simulink model "SingleTrack_RTW"  (Simulink 7.5)
settings: Solver=ode1  SolverMode=SingleTasking  StartTime=0.0  StopTime=inf  FixedStep=0.001  RelTol=1e-3
PreLoadFcn:
  | vehicle = 'Car'; if ~length(which('cmcmd')), cmenv; end
  | SingleTrack_RTW_bus;
  | SingleTrack_RTW_params;
InitFcn:
  | vehicle = 'Car'; if ~length(which('cmcmd')), cmenv; end
  | SingleTrack_RTW_bus;
  | SingleTrack_RTW_params;
values from neighbouring files (symbols this model uses):
  Car_Bdy1_mass = 650.0    (= 650)    [SingleTrack_RTW_params.m]    (also in UserVehicle_RTW_params.m)
  Car_Steering_i = 10.0    (= 10)    [SingleTrack_RTW_params.m]    (also in UserVehicle_RTW_params.m)
  Car_Whl_Radius = 0.31    [SingleTrack_RTW_params.m]    (also in UserVehicle_RTW_params.m)
  Car_WhlBaseF = 1.5    [SingleTrack_RTW_params.m]    (also in UserVehicle_RTW_params.m)
  Car_WhlBaseR = -1.5    [SingleTrack_RTW_params.m]    (also in UserVehicle_RTW_params.m)
  mEngineMax = 180    [SingleTrack_RTW_params.m]    (also in UserVehicle_RTW_params.m)
  PT_DL_iDiff = 4.1    [SingleTrack_RTW_params.m]    (also in UserVehicle_RTW_params.m)
  PT_GearBox_iForwardGears = [ 0 2.5 2.063 1.722 1.5 1.364 1.261]    [SingleTrack_RTW_params.m]    (also in UserVehicle_RTW_params.m)
libraries: CarMaker4SL x7
(part 3 of 3)

== system SingleTrack_RTW/SingleTrack/CreateBus Vhcl.Fr1/BdyFrame2Vhcl.Fr1A ==
  note: Translate pseudo BdyFrame interface to Vhcl.Fr1
  t_0 : Inport  OutDataType=sfix(16)  OutScaling=2^0
  v_0 : Inport  Port=2  OutDataType=sfix(16)  OutScaling=2^0
  a_0 : Inport  Port=3  OutDataType=sfix(16)  OutScaling=2^0
  omega_0 : Inport  Port=4  OutDataType=sfix(16)  OutScaling=2^0
  alpha_0 : Inport  Port=5  OutDataType=sfix(16)  OutScaling=2^0
  Tr2Fr0 : Inport  Port=6  OutDataType=sfix(16)  OutScaling=2^0
  Bus Creator : BusCreator  Inputs=24
  Demux{,1..3,5} (5 alike) : Demux  Outputs=3
  Demux4 : Demux  Outputs=9
  Vhcl.Fr1 : Outport  OutDataType=sfix(16)  OutScaling=2^0
  wires:
  Bus Creator/1 -> Vhcl.Fr1/1
  Demux/1 -> Bus Creator/1  "Vhcl Fr1 A_t_0 x"
  Demux/2 -> Bus Creator/2  "Vhcl Fr1A_t_0 y"
  Demux/3 -> Bus Creator/3  "Vhcl Fr1A_t_0 z"
  Demux1/1 -> Bus Creator/4  "Vhcl Fr1A_v_0 x"
  Demux1/2 -> Bus Creator/5  "Vhcl Fr1A_v_0 y"
  Demux1/3 -> Bus Creator/6  "Vhcl Fr1A_v_0 z"
  Demux2/1 -> Bus Creator/7  "Vhcl Fr1A_a_0 x"
  Demux2/2 -> Bus Creator/8  "Vhcl Fr1A_a_0 y"
  Demux2/3 -> Bus Creator/9  "Vhcl Fr1A_a_0 z"
  Demux3/1 -> Bus Creator/10  "Vhcl Fr1A_omega_0 x"
  Demux3/2 -> Bus Creator/11  "Vhcl Fr1A_omega_0 y"
  Demux3/3 -> Bus Creator/12  "Vhcl Fr1A_omega_0 z"
  Demux5/1 -> Bus Creator/13  "Vhcl Fr1A_alpha_0 x"
  Demux5/2 -> Bus Creator/14  "Vhcl Fr1A_alpha_0 y"
  Demux5/3 -> Bus Creator/15  "Vhcl Fr1A_alpha_0 z"
  Demux4/1 -> Bus Creator/16  "Vhcl Fr1A_Tr2Fr0 00"
  Demux4/2 -> Bus Creator/17  "Vhcl Fr1A_Tr2Fr0 01"
  Demux4/3 -> Bus Creator/18  "Vhcl Fr1A_Tr2Fr0 02"
  Demux4/4 -> Bus Creator/19  "Vhcl Fr1A_Tr2Fr0 10"
  Demux4/5 -> Bus Creator/20  "Vhcl Fr1A_Tr2Fr0 11"
  Demux4/6 -> Bus Creator/21  "Vhcl Fr1A_Tr2Fr0 12"
  Demux4/7 -> Bus Creator/22  "Vhcl Fr1A_Tr2Fr0 20"
  Demux4/8 -> Bus Creator/23  "Vhcl Fr1A_Tr2Fr0 21"
  Demux4/9 -> Bus Creator/24  "Vhcl Fr1A_Tr2Fr0 22"
  Tr2Fr0/1 -> Demux4/1
  alpha_0/1 -> Demux5/1
  omega_0/1 -> Demux3/1
  a_0/1 -> Demux2/1
  v_0/1 -> Demux1/1
  t_0/1 -> Demux/1

== system SingleTrack_RTW/SingleTrack/CreateBus Vhcl.Fr1/Tr2Fr0 ==
  Car : Inport  OutDataType=sfix(16)  OutScaling=2^0
  Bus Creator : BusCreator  Inputs=9
  Subsystem_00 : Subsystem
  Subsystem_01 : Subsystem
  Subsystem_02 : Subsystem
  Subsystem_10 : Subsystem
  Subsystem_11 : Subsystem
  Subsystem_12 : Subsystem
  Subsystem_20 : Subsystem
  Subsystem_21 : Subsystem
  Subsystem_22 : Subsystem
  sincos : Subsystem
  Tr2Fr0 : Outport  OutDataType=sfix(16)  OutScaling=2^0
  wires:
  Subsystem_12/1(Tr2Fr1_12) -> Bus Creator/6  "Tr2Fr1_12"
  Subsystem_11/1(Tr2Fr1_11) -> Bus Creator/5  "Tr2Fr1_11"
  Subsystem_02/1(Tr2Fr1_02) -> Bus Creator/3  "Tr2Fr0_02"
  Subsystem_01/1(Tr2Fr1_01) -> Bus Creator/2  "Tr2Fr0_01"
  Subsystem_22/1(Tr2Fr1_22) -> Bus Creator/9  "Tr2Fr0_22"
  Subsystem_21/1(Tr2Fr1_21) -> Bus Creator/8  "Tr2Fr0_21"
  Subsystem_20/1(Tr2Fr1_20) -> Bus Creator/7  "Tr2Fr0_20"
  Subsystem_10/1(Tr2Fr1_10) -> Bus Creator/4  "Tr2Fr0_10"
  Subsystem_00/1(Tr2Fr1_00) -> Bus Creator/1  "Tr2Fr0_00"
  Bus Creator/1 -> Tr2Fr0/1
  sincos/1(sincos) -> Subsystem_02/1(sincos), Subsystem_01/1(sincos), Subsystem_00/1(sincos), Subsystem_12/1(sincos), Subsystem_22/1(sincos), Subsystem_21/1(sincos), Subsystem_20/1(sincos), Subsystem_11/1(sincos), Subsystem_10/1(sincos)
  Car/1 -> sincos/1(Car)

== system SingleTrack_RTW/SingleTrack/CreateBus Vhcl.Fr1/a_0 ==
  Car : Inport  OutDataType=sfix(16)  OutScaling=2^0
  Tr2Fr0 : Inport  Port=2  OutDataType=sfix(16)  OutScaling=2^0
  Add : Sum  OutDataType=sfix(16)  OutScaling=2^-10
  Add1 : Sum  OutDataType=sfix(16)  OutScaling=2^-10
  Add2 : Sum  OutDataType=sfix(16)  OutScaling=2^-10
  Bus Selector1 : BusSelector  OutputSignals=Car_ax_1,Car_ay_1
  Bus Selector2 : BusSelector  OutputSignals=Tr2Fr0_00,Tr2Fr0_01,Tr2Fr0_10,Tr2Fr1_11,Tr2Fr0_20,Tr2Fr0_21
  Mux1 : Mux  Inputs=3
  Product{,1..5} (6 alike) : Product  OutDataType=sfix(16)  OutScaling=2^0  RndMeth=Zero
  a_0 : Outport  OutDataType=sfix(16)  OutScaling=2^0
  wires:
  Bus Selector2/5 -> Product5/2  "<Tr2Fr0_20>"
  Bus Selector2/6 -> Product4/2  "<Tr2Fr0_21>"
  Add2/1 -> Mux1/3
  Product4/1 -> Add2/2
  Product5/1 -> Add2/1
  Bus Selector2/4 -> Product2/2  "<Tr2Fr1_11>"
  Bus Selector2/3 -> Product3/2  "<Tr2Fr0_10>"
  Add1/1 -> Mux1/2
  Bus Selector2/2 -> Product/2  "<Tr2Fr0_01>"
  Bus Selector2/1 -> Product1/2  "<Tr2Fr0_00>"
  Product2/1 -> Add1/2
  Product3/1 -> Add1/1
  Add/1 -> Mux1/1
  Product/1 -> Add/2
  Product1/1 -> Add/1
  Bus Selector1/1 -> Product5/1, Product3/1, Product1/1  "<Car_ax_1>"
  Bus Selector1/2 -> Product4/1, Product2/1, Product/1  "<Car_ay_1>"
  Tr2Fr0/1 -> Bus Selector2/1
  Car/1 -> Bus Selector1/1
  Mux1/1 -> a_0/1

== system SingleTrack_RTW/SingleTrack/CreateBus Vhcl.Fr1/t_0 ==
  Car : Inport  OutDataType=sfix(16)  OutScaling=2^0
  Bus Selector : BusSelector  OutputSignals=Car_x,Car_y,Road_Fr1_z
  Mux : Mux  Inputs=3
  t_0 : Outport  OutDataType=sfix(16)  OutScaling=2^0
  wires:
  Mux/1 -> t_0/1
  Car/1 -> Bus Selector/1
  Bus Selector/3 -> Mux/3  "<Road_Fr1_z>"
  Bus Selector/2 -> Mux/2  "<Car_y>"
  Bus Selector/1 -> Mux/1  "<Car_x>"

== system SingleTrack_RTW/SingleTrack/CreateBus Vhcl.Fr1/v_0 ==
  Car : Inport  OutDataType=sfix(16)  OutScaling=2^0
  Tr2Fr0 : Inport  Port=2  OutDataType=sfix(16)  OutScaling=2^0
  Bus Selector1 : BusSelector  OutputSignals=Car_vx_1
  Bus Selector2 : BusSelector  OutputSignals=Tr2Fr0_00,Tr2Fr0_10,Tr2Fr0_20
  Mux1 : Mux  Inputs=3
  Product : Product  OutDataType=sfix(16)  OutScaling=2^0  RndMeth=Zero
  Product1 : Product  OutDataType=sfix(16)  OutScaling=2^0  RndMeth=Zero
  Product2 : Product  OutDataType=sfix(16)  OutScaling=2^0  RndMeth=Zero
  v_0 : Outport  OutDataType=sfix(16)  OutScaling=2^0
  wires:
  Product2/1 -> Mux1/3
  Product1/1 -> Mux1/2
  Product/1 -> Mux1/1
  Bus Selector1/1 -> Product2/1, Product1/1, Product/1  "<Car_vx_1>"
  Bus Selector2/3 -> Product2/2  "<Tr2Fr0_20>"
  Bus Selector2/2 -> Product1/2  "<Tr2Fr0_10>"
  Bus Selector2/1 -> Product/2  "<Tr2Fr0_00>"
  Tr2Fr0/1 -> Bus Selector2/1
  Mux1/1 -> v_0/1
  Car/1 -> Bus Selector1/1

== system SingleTrack_RTW/SingleTrack/single-track mass point model/Car.v_1 ==
  ax : Inport
  Constant1 : Constant  Value=0.1  OutDataType=sfix(16)  OutScaling=2^0
  PassIfSim : Subsystem
  Read CM Parameter : CarMaker4SL/Read CM Parameter  xfile=Testrun  xkey=DrivMan.Init.Velocity  xnout=1  xdefaults=0  xmuxed=on
  kmh2ms : Gain  Gain=1000/3600  ParameterDataType=sfix(16)  ParameterScaling=2^0  OutDataType=sfix(16)  OutScaling=2^0  OutDataTypeStr=Inherit: Inherit via back propagation  SaturateOnIntegerOverflow=on  ParamDataTypeStr=Inherit: Same as input
  vMin : MinMax  Function=max  Inputs=2  OutDataType=sfix(16)  OutScaling=2^0  SaturateOnIntegerOverflow=on  InputSameDT=on
  v_dot * dt : Integrator  ExternalReset=level  InitialConditionSource=external  InitialCondition=22.222
  v_1 : Outport  PortDimensions=1
  wires:
  PassIfSim/1(Out1) -> v_dot * dt/1
  ax/1 -> PassIfSim/1(In1)
  v_dot * dt/1 -> v_1/1
  vMin/1 -> v_dot * dt/3
  [TRStart] -> v_dot * dt/2
  Constant1/1 -> vMin/1
  kmh2ms/1 -> vMin/2
  Read CM Parameter/1 -> kmh2ms/1

== system SingleTrack_RTW/SingleTrack/single-track mass point model/PassIfSim ==
  note: Output original value only when simulating,
      | and zero during pre- or postprocessing.
  In1 : Inport  OutDataType=sfix(16)  OutScaling=2^0
  "   " : Product  OutDataType=sfix(16)  OutScaling=2^0  SaturateOnIntegerOverflow=on  InputSameDT=on  OutDataTypeStr=Inherit: Same as first input
  Data Type Conversion : DataTypeConversion  OutDataType=sfix(16)  OutScaling=2^0
  Out1 : Outport  OutDataType=sfix(16)  OutScaling=2^0
  wires:
  In1/1 -> "   "/1
  Data Type Conversion/1 -> "   "/2
  "   "/1 -> Out1/1
  [TRSim] -> Data Type Conversion/1

== system SingleTrack_RTW/SingleTrack/single-track mass point model/PassIfSim1 ==
  note: Output original value only when simulating,
      | and zero during pre- or postprocessing.
  In1 : Inport  OutDataType=sfix(16)  OutScaling=2^0
  "   " : Product  OutDataType=sfix(16)  OutScaling=2^0  SaturateOnIntegerOverflow=on  InputSameDT=on  OutDataTypeStr=Inherit: Same as first input
  Data Type Conversion : DataTypeConversion  OutDataType=sfix(16)  OutScaling=2^0
  Out1 : Outport  OutDataType=sfix(16)  OutScaling=2^0
  wires:
  In1/1 -> "   "/1
  Data Type Conversion/1 -> "   "/2
  "   "/1 -> Out1/1
  [TRSim] -> Data Type Conversion/1

== system SingleTrack_RTW/SingleTrack/single-track mass point model/PassIfSim2 ==
  note: Output original value only when simulating,
      | and zero during pre- or postprocessing.
  In1 : Inport  OutDataType=sfix(16)  OutScaling=2^0
  "   " : Product  OutDataType=sfix(16)  OutScaling=2^0  SaturateOnIntegerOverflow=on  InputSameDT=on  OutDataTypeStr=Inherit: Same as first input
  Data Type Conversion : DataTypeConversion  OutDataType=sfix(16)  OutScaling=2^0
  Out1 : Outport  OutDataType=sfix(16)  OutScaling=2^0
  wires:
  In1/1 -> "   "/1
  Data Type Conversion/1 -> "   "/2
  "   "/1 -> Out1/1
  [TRSim] -> Data Type Conversion/1

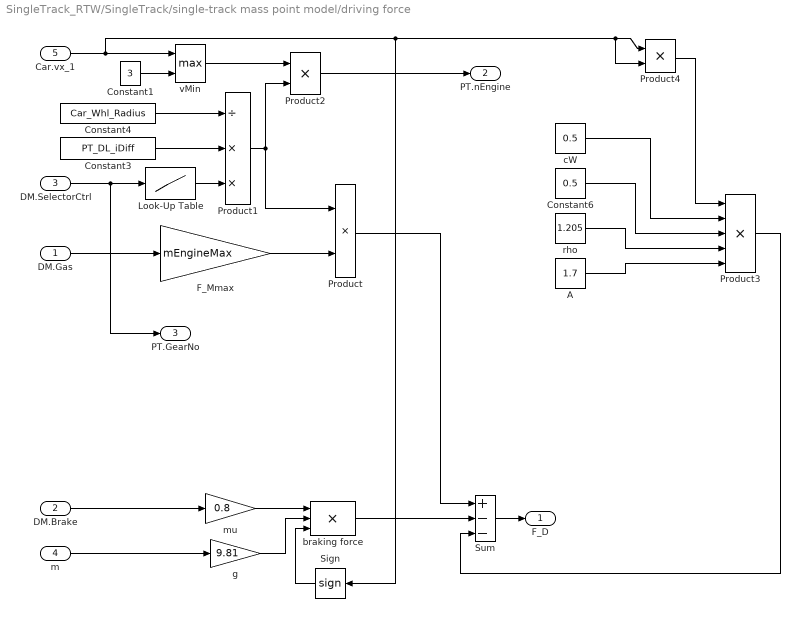
== system SingleTrack_RTW/SingleTrack/single-track mass point model/driving force ==
  DM.Gas : Inport  OutDataType=sfix(16)  OutScaling=2^0
  DM.Brake : Inport  Port=2  OutDataType=sfix(16)  OutScaling=2^0
  DM.SelectorCtrl : Inport  Port=3  OutDataType=sfix(16)  OutScaling=2^0
  m : Inport  Port=4  OutDataType=sfix(16)  OutScaling=2^0
  Car.vx_1 : Inport  Port=5  OutDataType=sfix(16)  OutScaling=2^0
  A : Constant  Value=1.7  OutDataType=sfix(16)  OutScaling=2^0
  Constant1 : Constant  Value=3  OutDataType=sfix(16)  OutScaling=2^0
  Constant3 : Constant  Value=PT_DL_iDiff  OutDataType=sfix(16)  OutScaling=2^0
  Constant4 : Constant  Value=Car_Whl_Radius  OutDataType=sfix(16)  OutScaling=2^0
  Constant6 : Constant  Value=0.5  OutDataType=sfix(16)  OutScaling=2^0
  "F_Mmax " : Gain  Gain=mEngineMax  ParameterDataType=sfix(16)  ParameterScaling=2^0  OutDataType=sfix(16)  OutScaling=2^0  SaturateOnIntegerOverflow=on  OutDataTypeStr=Inherit: Same as input  ParamDataTypeStr=Inherit: Same as input
  Look-Up Table : Lookup  InputValues=[0 1 2 3 4 5 6]  Table=PT_GearBox_iForwardGears  LookUpMeth=Interpolation-Use End Values  OutDataType=sfix(16)  OutScaling=2^0  SaturateOnIntegerOverflow=on
  Product : Product  Inputs=**  OutDataType=sfix(16)  OutScaling=2^0  SaturateOnIntegerOverflow=on  InputSameDT=on  OutDataTypeStr=Inherit: Same as first input
  Product1 : Product  Inputs=/**  OutDataType=sfix(16)  OutScaling=2^0  SaturateOnIntegerOverflow=on  InputSameDT=on  OutDataTypeStr=Inherit: Same as first input
  Product2 : Product  OutDataType=sfix(16)  OutScaling=2^0  SaturateOnIntegerOverflow=on  InputSameDT=on  OutDataTypeStr=Inherit: Same as first input
  Product3 : Product  Inputs=5  OutDataType=sfix(16)  OutScaling=2^0  SaturateOnIntegerOverflow=on  InputSameDT=on  OutDataTypeStr=Inherit: Same as first input
  Product4 : Product  OutDataType=sfix(16)  OutScaling=2^0  SaturateOnIntegerOverflow=on  InputSameDT=on  OutDataTypeStr=Inherit: Same as first input
  Sign : Signum
  Sum : Sum  Inputs=+--  OutDataType=sfix(16)  OutScaling=2^0  SaturateOnIntegerOverflow=on  InputSameDT=on  OutDataTypeStr=Inherit: Same as first input
  braking force : Product  Inputs=3  OutDataType=sfix(16)  OutScaling=2^0  SaturateOnIntegerOverflow=on  InputSameDT=on  OutDataTypeStr=Inherit: Same as first input
  cW : Constant  Value=0.5  OutDataType=sfix(16)  OutScaling=2^0
  g : Gain  Gain=9.81  ParameterDataType=sfix(16)  ParameterScaling=2^0  OutDataType=sfix(16)  OutScaling=2^0  SaturateOnIntegerOverflow=on  OutDataTypeStr=Inherit: Same as input  ParamDataTypeStr=Inherit: Same as input
  mu : Gain  Gain=0.8  ParameterDataType=sfix(16)  ParameterScaling=2^0  OutDataType=sfix(16)  OutScaling=2^0  SaturateOnIntegerOverflow=on  OutDataTypeStr=Inherit: Same as input  ParamDataTypeStr=Inherit: Same as input
  rho : Constant  Value=1.205  OutDataType=sfix(16)  OutScaling=2^0
  vMin : MinMax  Function=max  Inputs=2  OutDataType=sfix(16)  OutScaling=2^0  SaturateOnIntegerOverflow=on  InputSameDT=on
  F_D : Outport  OutDataType=sfix(16)  OutScaling=2^0
  PT.nEngine : Outport  Port=2  OutDataType=sfix(16)  OutScaling=2^0
  PT.GearNo : Outport  Port=3  OutDataType=sfix(16)  OutScaling=2^0
  wires:
  vMin/1 -> Product2/1
  Car.vx_1/1 -> vMin/1, Product4/1, Product4/2, Sign/1
  Constant1/1 -> vMin/2
  DM.Brake/1 -> mu/1
  "F_Mmax "/1 -> Product/2
  Product2/1 -> PT.nEngine/1
  Look-Up Table/1 -> Product1/3
  Product1/1 -> Product/1, Product2/2
  Constant4/1 -> Product1/1
  Constant3/1 -> Product1/2
  Product/1 -> Sum/1
  Sum/1 -> F_D/1
  braking force/1 -> Sum/2
  g/1 -> braking force/2
  m/1 -> g/1
  mu/1 -> braking force/1
  DM.Gas/1 -> "F_Mmax "/1
  A/1 -> Product3/5
  rho/1 -> Product3/4
  Constant6/1 -> Product3/3
  cW/1 -> Product3/2
  Product4/1 -> Product3/1
  Product3/1 -> Sum/3
  Sign/1 -> braking force/3
  DM.SelectorCtrl/1 -> Look-Up Table/1, PT.GearNo/1

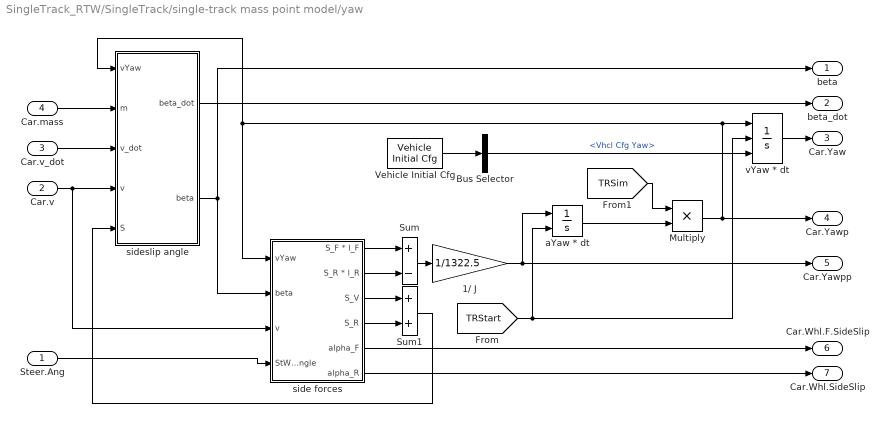
== system SingleTrack_RTW/SingleTrack/single-track mass point model/yaw ==
  Steer.Ang : Inport  OutDataType=sfix(16)  OutScaling=2^0
  Car.v : Inport  Port=2  OutDataType=sfix(16)  OutScaling=2^0
  Car.v_dot : Inport  Port=3  OutDataType=sfix(16)  OutScaling=2^0
  Car.mass : Inport  Port=4  OutDataType=sfix(16)  OutScaling=2^0
  1/ J : Gain  Gain=1/1322.5  ParameterDataType=sfix(16)  ParameterScaling=2^0  OutDataType=sfix(16)  OutScaling=2^0  SaturateOnIntegerOverflow=on  OutDataTypeStr=Inherit: Same as input  ParamDataTypeStr=Inherit: Same as input
  Bus Selector : BusSelector  OutputSignals=Vhcl Cfg Yaw
  Multiply : Product  Inputs=**  OutDataTypeMode=double  OutDataType=sfix(16)  OutScaling=2^-10  OutDataTypeStr=double
  Sum : Sum  Inputs=+-  OutDataType=sfix(16)  OutScaling=2^0  SaturateOnIntegerOverflow=on  InputSameDT=on  OutDataTypeStr=Inherit: Same as first input
  Sum1 : Sum  OutDataType=sfix(16)  OutScaling=2^0  SaturateOnIntegerOverflow=on  InputSameDT=on  OutDataTypeStr=Inherit: Same as first input
  Vehicle Initial Cfg : CarMaker4SL/Vehicle Initial Cfg  SystemSampleTime=-1
  aYaw * dt : Integrator  ExternalReset=level
  side forces : Subsystem
  sideslip angle : Subsystem
  vYaw * dt : Integrator  ExternalReset=level  InitialConditionSource=external
  beta : Outport  OutDataType=sfix(16)  OutScaling=2^0
  beta_dot : Outport  Port=2  OutDataType=sfix(16)  OutScaling=2^0
  Car.Yaw : Outport  Port=3  OutDataType=sfix(16)  OutScaling=2^0
  Car.Yawp : Outport  Port=4  OutDataType=sfix(16)  OutScaling=2^0
  Car.Yawpp : Outport  Port=5  OutDataType=sfix(16)  OutScaling=2^0
  Car.Whl.F.SideSlip : Outport  Port=6  OutDataType=sfix(16)  OutScaling=2^0
  Car.Whl.SideSlip : Outport  Port=7  OutDataType=sfix(16)  OutScaling=2^0
  wires:
  Bus Selector/1 -> vYaw * dt/3  "<Vhcl Cfg Yaw>"
  side forces/6(alpha_R) -> Car.Whl.SideSlip/1
  side forces/5(alpha_F) -> Car.Whl.F.SideSlip/1
  sideslip angle/1(beta_dot) -> beta_dot/1
  Steer.Ang/1 -> side forces/4(StWhlAngle)
  sideslip angle/2(beta) -> beta/1, side forces/2(beta)
  Car.mass/1 -> sideslip angle/2(m)
  Car.v_dot/1 -> sideslip angle/3(v_dot)
  Sum1/1 -> sideslip angle/5(S)
  Sum/1 -> 1/ J/1
  side forces/1(S_F * l_F) -> Sum/1
  side forces/2(S_R * l_R) -> Sum/2
  1/ J/1 -> Car.Yawpp/1, aYaw * dt/1
  side forces/3(S_V) -> Sum1/1
  side forces/4(S_R) -> Sum1/2
  Car.v/1 -> sideslip angle/4(v), side forces/3(v)
  vYaw * dt/1 -> Car.Yaw/1
  Multiply/1 -> side forces/1(vYaw), sideslip angle/1(vYaw), vYaw * dt/1, Car.Yawp/1
  [TRStart] -> vYaw * dt/2, aYaw * dt/2
  aYaw * dt/1 -> Multiply/2
  [TRSim] -> Multiply/1
  Vehicle Initial Cfg/1 -> Bus Selector/1

== system SingleTrack_RTW/SingleTrack/CreateBus Vhcl.Fr1/Tr2Fr0/Subsystem_00 ==
  sincos : Inport  OutDataType=sfix(16)  OutScaling=2^0
  Bus Selector : BusSelector  OutputSignals=cry,crz
  Product : Product  OutDataType=sfix(16)  OutScaling=2^0  RndMeth=Zero
  Tr2Fr1_00 : Outport  OutDataType=sfix(16)  OutScaling=2^0
  wires:
  Bus Selector/2 -> Product/2  "<crz>"
  Bus Selector/1 -> Product/1  "<cry>"
  Product/1 -> Tr2Fr1_00/1
  sincos/1 -> Bus Selector/1

== system SingleTrack_RTW/SingleTrack/CreateBus Vhcl.Fr1/Tr2Fr0/Subsystem_01 ==
  sincos : Inport  OutDataType=sfix(16)  OutScaling=2^0
  Add : Sum  Inputs=+-  OutDataType=sfix(16)  OutScaling=2^-10
  Bus Selector : BusSelector  OutputSignals=srx,sry,crz,crx,srz
  Product : Product  Inputs=3  OutDataType=sfix(16)  OutScaling=2^0  RndMeth=Zero
  Product1 : Product  OutDataType=sfix(16)  OutScaling=2^0  RndMeth=Zero
  Tr2Fr1_01 : Outport  OutDataType=sfix(16)  OutScaling=2^0
  wires:
  Bus Selector/5 -> Product1/2  "<srz>"
  Bus Selector/4 -> Product1/1  "<crx>"
  Bus Selector/3 -> Product/3  "<crz>"
  Bus Selector/2 -> Product/2  "<sry>"
  Bus Selector/1 -> Product/1  "<srx>"
  Add/1 -> Tr2Fr1_01/1
  Product1/1 -> Add/2
  Product/1 -> Add/1
  sincos/1 -> Bus Selector/1

== system SingleTrack_RTW/SingleTrack/CreateBus Vhcl.Fr1/Tr2Fr0/Subsystem_02 ==
  sincos : Inport  OutDataType=sfix(16)  OutScaling=2^0
  Add : Sum  OutDataType=sfix(16)  OutScaling=2^-10
  Bus Selector : BusSelector  OutputSignals=crx,sry,crz,srx,srz
  Product : Product  Inputs=3  OutDataType=sfix(16)  OutScaling=2^0  RndMeth=Zero
  Product1 : Product  OutDataType=sfix(16)  OutScaling=2^0  RndMeth=Zero
  Tr2Fr1_02 : Outport  OutDataType=sfix(16)  OutScaling=2^0
  wires:
  Bus Selector/4 -> Product1/1  "<srx>"
  Bus Selector/5 -> Product1/2  "<srz>"
  Bus Selector/3 -> Product/3  "<crz>"
  Bus Selector/2 -> Product/2  "<sry>"
  Bus Selector/1 -> Product/1  "<crx>"
  sincos/1 -> Bus Selector/1
  Product/1 -> Add/1
  Product1/1 -> Add/2
  Add/1 -> Tr2Fr1_02/1

== system SingleTrack_RTW/SingleTrack/CreateBus Vhcl.Fr1/Tr2Fr0/Subsystem_10 ==
  sincos : Inport  OutDataType=sfix(16)  OutScaling=2^0
  Bus Selector : BusSelector  OutputSignals=cry,srz
  Product : Product  OutDataType=sfix(16)  OutScaling=2^0  RndMeth=Zero
  Tr2Fr1_10 : Outport  OutDataType=sfix(16)  OutScaling=2^0
  wires:
  sincos/1 -> Bus Selector/1
  Product/1 -> Tr2Fr1_10/1
  Bus Selector/1 -> Product/1  "<cry>"
  Bus Selector/2 -> Product/2  "<srz>"

== system SingleTrack_RTW/SingleTrack/CreateBus Vhcl.Fr1/Tr2Fr0/Subsystem_11 ==
  sincos : Inport  OutDataType=sfix(16)  OutScaling=2^0
  Add : Sum  OutDataType=sfix(16)  OutScaling=2^-10
  Bus Selector : BusSelector  OutputSignals=srx,sry,srz,crx,crz
  Product : Product  Inputs=3  OutDataType=sfix(16)  OutScaling=2^0  RndMeth=Zero
  Product1 : Product  OutDataType=sfix(16)  OutScaling=2^0  RndMeth=Zero
  Tr2Fr1_11 : Outport  OutDataType=sfix(16)  OutScaling=2^0
  wires:
  Bus Selector/4 -> Product1/1  "<crx>"
  Bus Selector/5 -> Product1/2  "<crz>"
  Bus Selector/3 -> Product/3  "<srz>"
  Bus Selector/2 -> Product/2  "<sry>"
  Bus Selector/1 -> Product/1  "<srx>"
  Add/1 -> Tr2Fr1_11/1
  Product1/1 -> Add/2
  Product/1 -> Add/1
  sincos/1 -> Bus Selector/1

== system SingleTrack_RTW/SingleTrack/CreateBus Vhcl.Fr1/Tr2Fr0/Subsystem_12 ==
  sincos : Inport  OutDataType=sfix(16)  OutScaling=2^0
  Add : Sum  Inputs=+-  OutDataType=sfix(16)  OutScaling=2^-10
  Bus Selector : BusSelector  OutputSignals=crx,sry,srz,srx,crz
  Product : Product  Inputs=3  OutDataType=sfix(16)  OutScaling=2^0  RndMeth=Zero
  Product1 : Product  OutDataType=sfix(16)  OutScaling=2^0  RndMeth=Zero
  Tr2Fr1_12 : Outport  OutDataType=sfix(16)  OutScaling=2^0
  wires:
  Bus Selector/4 -> Product1/1  "<srx>"
  Bus Selector/5 -> Product1/2  "<crz>"
  Bus Selector/3 -> Product/3  "<srz>"
  Bus Selector/2 -> Product/2  "<sry>"
  Bus Selector/1 -> Product/1  "<crx>"
  sincos/1 -> Bus Selector/1
  Product/1 -> Add/1
  Product1/1 -> Add/2
  Add/1 -> Tr2Fr1_12/1

== system SingleTrack_RTW/SingleTrack/CreateBus Vhcl.Fr1/Tr2Fr0/Subsystem_20 ==
  sincos : Inport  OutDataType=sfix(16)  OutScaling=2^0
  Bus Selector : BusSelector  OutputSignals=sry
  Gain : Gain  Gain=-1  ParameterDataType=sfix(16)  ParameterScaling=2^0  OutDataType=sfix(16)  OutScaling=2^0
  Tr2Fr1_20 : Outport  OutDataType=sfix(16)  OutScaling=2^0
  wires:
  Bus Selector/1 -> Gain/1  "<sry>"
  Gain/1 -> Tr2Fr1_20/1
  sincos/1 -> Bus Selector/1

== system SingleTrack_RTW/SingleTrack/CreateBus Vhcl.Fr1/Tr2Fr0/Subsystem_21 ==
  sincos : Inport  OutDataType=sfix(16)  OutScaling=2^0
  Bus Selector : BusSelector  OutputSignals=srx,cry
  Product : Product  OutDataType=sfix(16)  OutScaling=2^0  RndMeth=Zero
  Tr2Fr1_21 : Outport  OutDataType=sfix(16)  OutScaling=2^0
  wires:
  Bus Selector/2 -> Product/2  "<cry>"
  Bus Selector/1 -> Product/1  "<srx>"
  Product/1 -> Tr2Fr1_21/1
  sincos/1 -> Bus Selector/1

== system SingleTrack_RTW/SingleTrack/CreateBus Vhcl.Fr1/Tr2Fr0/Subsystem_22 ==
  sincos : Inport  OutDataType=sfix(16)  OutScaling=2^0
  Bus Selector : BusSelector  OutputSignals=crx,cry
  Product : Product  OutDataType=sfix(16)  OutScaling=2^0  RndMeth=Zero
  Tr2Fr1_22 : Outport  OutDataType=sfix(16)  OutScaling=2^0
  wires:
  Bus Selector/2 -> Product/2  "<cry>"
  Bus Selector/1 -> Product/1  "<crx>"
  sincos/1 -> Bus Selector/1
  Product/1 -> Tr2Fr1_22/1

== system SingleTrack_RTW/SingleTrack/CreateBus Vhcl.Fr1/Tr2Fr0/sincos ==
  Car : Inport  OutDataType=sfix(16)  OutScaling=2^0
  Bus Creator : BusCreator  Inputs=6
  Bus Selector : BusSelector  OutputSignals=Road_Fr1_rx,Road_Fr1_ry,Car_Yaw
  Trigonometric Function : Trigonometry
  Trigonometric Function1 : Trigonometry  Operator=cos
  Trigonometric Function2 : Trigonometry
  Trigonometric Function3 : Trigonometry
  Trigonometric Function4 : Trigonometry  Operator=cos
  Trigonometric Function5 : Trigonometry  Operator=cos
  sincos : Outport  OutDataType=sfix(16)  OutScaling=2^0
  wires:
  Bus Creator/1 -> sincos/1
  Trigonometric Function/1 -> Bus Creator/1  "srx"
  Trigonometric Function3/1 -> Bus Creator/2  "sry"
  Trigonometric Function2/1 -> Bus Creator/3  "srz"
  Trigonometric Function1/1 -> Bus Creator/4  "crx"
  Trigonometric Function4/1 -> Bus Creator/5  "cry"
  Trigonometric Function5/1 -> Bus Creator/6  "crz"
  Car/1 -> Bus Selector/1
  Bus Selector/3 -> Trigonometric Function5/1, Trigonometric Function2/1  "<Car_Yaw>"
  Bus Selector/2 -> Trigonometric Function4/1, Trigonometric Function3/1  "<Road_Fr1_ry>"
  Bus Selector/1 -> Trigonometric Function1/1, Trigonometric Function/1  "<Road_Fr1_rx>"

== system SingleTrack_RTW/SingleTrack/single-track mass point model/Car.v_1/PassIfSim ==
  note: Output original value only when simulating,
      | and zero during pre- or postprocessing.
  In1 : Inport  OutDataType=sfix(16)  OutScaling=2^0
  "   " : Product  OutDataType=sfix(16)  OutScaling=2^0  SaturateOnIntegerOverflow=on  InputSameDT=on  OutDataTypeStr=Inherit: Same as first input
  Data Type Conversion : DataTypeConversion  OutDataType=sfix(16)  OutScaling=2^0
  Out1 : Outport  OutDataType=sfix(16)  OutScaling=2^0
  wires:
  In1/1 -> "   "/1
  Data Type Conversion/1 -> "   "/2
  "   "/1 -> Out1/1
  [TRSim] -> Data Type Conversion/1

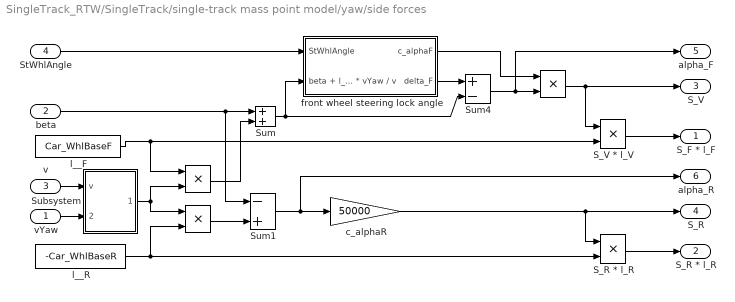
== system SingleTrack_RTW/SingleTrack/single-track mass point model/yaw/side forces ==
  vYaw : Inport  OutDataType=sfix(16)  OutScaling=2^0
  beta : Inport  Port=2  OutDataType=sfix(16)  OutScaling=2^0
  v : Inport  Port=3  OutDataType=sfix(16)  OutScaling=2^0
  StWhlAngle : Inport  Port=4  OutDataType=sfix(16)  OutScaling=2^0
  " " : Product  OutDataType=sfix(16)  OutScaling=2^0  SaturateOnIntegerOverflow=on  InputSameDT=on  OutDataTypeStr=Inherit: Same as first input
  "  " : Product  OutDataType=sfix(16)  OutScaling=2^0  SaturateOnIntegerOverflow=on  InputSameDT=on  OutDataTypeStr=Inherit: Same as first input
  "            " : Product  OutDataType=sfix(16)  OutScaling=2^0  SaturateOnIntegerOverflow=on  InputSameDT=on  OutDataTypeStr=Inherit: Same as first input
  "S_R * l_R " : Product  OutDataType=sfix(16)  OutScaling=2^0  SaturateOnIntegerOverflow=on  InputSameDT=on  OutDataTypeStr=Inherit: Same as first input
  "S_V * l_V " : Product  OutDataType=sfix(16)  OutScaling=2^0  SaturateOnIntegerOverflow=on  InputSameDT=on  OutDataTypeStr=Inherit: Same as first input
  Subsystem : Subsystem
  Sum : Sum  OutDataType=sfix(16)  OutScaling=2^0  SaturateOnIntegerOverflow=on  InputSameDT=on  OutDataTypeStr=Inherit: Same as first input
  Sum1 : Sum  Inputs=-+  OutDataType=sfix(16)  OutScaling=2^0  SaturateOnIntegerOverflow=on  InputSameDT=on  OutDataTypeStr=Inherit: Same as first input
  Sum4 : Sum  Inputs=+-  OutDataType=sfix(16)  OutScaling=2^0  SaturateOnIntegerOverflow=on  InputSameDT=on  OutDataTypeStr=Inherit: Same as first input
  c_alphaR : Gain  Gain=50000  ParameterDataType=sfix(16)  ParameterScaling=2^0  OutDataType=sfix(16)  OutScaling=2^0  SaturateOnIntegerOverflow=on  OutDataTypeStr=Inherit: Same as input  ParamDataTypeStr=Inherit: Same as input
  front wheel steering lock angle : Subsystem
  l__F : Constant  Value=Car_WhlBaseF  OutDataType=sfix(16)  OutScaling=2^0
  l__R : Constant  Value=-Car_WhlBaseR  OutDataType=sfix(16)  OutScaling=2^0
  S_F * l_F : Outport  OutDataType=sfix(16)  OutScaling=2^0
  S_R * l_R : Outport  Port=2  OutDataType=sfix(16)  OutScaling=2^0
  S_V : Outport  Port=3  OutDataType=sfix(16)  OutScaling=2^0
  S_R : Outport  Port=4  OutDataType=sfix(16)  OutScaling=2^0
  alpha_F : Outport  Port=5  OutDataType=sfix(16)  OutScaling=2^0
  alpha_R : Outport  Port=6  OutDataType=sfix(16)  OutScaling=2^0
  wires:
  front wheel steering lock angle/1(c_alphaF) -> "            "/1
  StWhlAngle/1 -> front wheel steering lock angle/1(StWhlAngle)
  "S_R * l_R "/1 -> S_R * l_R/1
  Sum4/1 -> alpha_F/1, "            "/2
  front wheel steering lock angle/2(delta_F) -> Sum4/1
  Sum/1 -> front wheel steering lock angle/2(beta + l_F * vYaw / v), Sum4/2
  v/1 -> Subsystem/1(v)
  vYaw/1 -> Subsystem/2(vYaw)
  "S_V * l_V "/1 -> S_F * l_F/1
  "            "/1 -> S_V/1, "S_V * l_V "/1
  c_alphaR/1 -> S_R/1, "S_R * l_R "/1
  Sum1/1 -> alpha_R/1, c_alphaR/1
  "  "/1 -> Sum/2
  " "/1 -> Sum1/2
  l__R/1 -> "S_R * l_R "/2, " "/2
  Subsystem/1(vYaw/v) -> "  "/2, " "/1
  l__F/1 -> "S_V * l_V "/2, "  "/1
  beta/1 -> Sum/1, Sum1/1

== system SingleTrack_RTW/SingleTrack/single-track mass point model/yaw/sideslip angle ==
  vYaw : Inport  OutDataType=sfix(16)  OutScaling=2^0
  m : Inport  Port=2  OutDataType=sfix(16)  OutScaling=2^0
  v_dot : Inport  Port=3  OutDataType=sfix(16)  OutScaling=2^0
  v : Inport  Port=4  OutDataType=sfix(16)  OutScaling=2^0
  S : Inport  Port=5  OutDataType=sfix(16)  OutScaling=2^0
  " " : Product  Inputs=*/  OutDataType=sfix(16)  OutScaling=2^0  SaturateOnIntegerOverflow=on  InputSameDT=on  OutDataTypeStr=Inherit: Same as first input
  "  " : Product  OutDataType=sfix(16)  OutScaling=2^0  SaturateOnIntegerOverflow=on  InputSameDT=on  OutDataTypeStr=Inherit: Same as first input
  Subsystem : Subsystem
  Sum2 : Sum  Inputs=+-  OutDataType=sfix(16)  OutScaling=2^0  SaturateOnIntegerOverflow=on  InputSameDT=on  OutDataTypeStr=Inherit: Same as first input
  beta_dot * dt : Integrator  ExternalReset=level
  beta_dot : Outport  OutDataType=sfix(16)  OutScaling=2^0
  beta : Outport  Port=2  OutDataType=sfix(16)  OutScaling=2^0
  wires:
  v/1 -> Subsystem/2(v)
  Subsystem/1(Out1) -> beta_dot/1, beta_dot * dt/1
  vYaw/1 -> Subsystem/1(vYaw)
  Sum2/1 -> Subsystem/3(In3)
  "  "/1 -> Sum2/2
  m/1 -> " "/2
  v_dot/1 -> "  "/1
  " "/1 -> Sum2/1
  S/1 -> " "/1
  beta_dot * dt/1 -> "  "/2, beta/1
  [TRStart] -> beta_dot * dt/2

== system SingleTrack_RTW/SingleTrack/single-track mass point model/yaw/side forces/Subsystem ==
  v : Inport
  vYaw : Inport  Port=2
  If : If  IfExpression=u1 > 0.1 | u1 < -0.1
  If Action Subsystem : Subsystem  TreatAsAtomicUnit=on
  If Action Subsystem1 : Subsystem  TreatAsAtomicUnit=on
  Merge : Merge  InitialOutput=0
  vYaw/v : Outport
  wires:
  v/1 -> If Action Subsystem/1(v), If/1
  vYaw/1 -> If Action Subsystem/2(vYaw)
  If/1 -> If Action Subsystem/Action
  If/2 -> If Action Subsystem1/Action
  Merge/1 -> vYaw/v/1
  If Action Subsystem/1(Out1) -> Merge/1
  If Action Subsystem1/1(Out1) -> Merge/2

== system SingleTrack_RTW/SingleTrack/single-track mass point model/yaw/side forces/front wheel steering lock angle ==
  StWhlAngle : Inport  OutDataType=sfix(16)  OutScaling=2^0
  beta + l_F * vYaw / v : Inport  Port=2  OutDataType=sfix(16)  OutScaling=2^0
  "   " : Product  OutDataType=sfix(16)  OutScaling=2^0  SaturateOnIntegerOverflow=on  InputSameDT=on  OutDataTypeStr=Inherit: Same as first input
  "     " : Constant  OutDataType=sfix(16)  OutScaling=2^0
  "      " : Product  Inputs=*/  OutDataType=sfix(16)  OutScaling=2^0  SaturateOnIntegerOverflow=on  InputSameDT=on  OutDataTypeStr=Inherit: Same as first input
  "       " : Product  Inputs=*/*  OutDataType=sfix(16)  OutScaling=2^0  SaturateOnIntegerOverflow=on  InputSameDT=on  OutDataTypeStr=Inherit: Same as first input
  1/ i_S : Gain  Gain=1/Car_Steering_i  ParameterDataType=sfix(16)  ParameterScaling=2^0  OutDataType=sfix(16)  OutScaling=2^0  SaturateOnIntegerOverflow=on  OutDataTypeStr=Inherit: Same as input  ParamDataTypeStr=Inherit: Same as input
  C_S : Constant  Value=10000  OutDataType=sfix(16)  OutScaling=2^0
  Sum2 : Sum  OutDataType=sfix(16)  OutScaling=2^0  SaturateOnIntegerOverflow=on  InputSameDT=on  OutDataTypeStr=Inherit: Same as first input
  Sum3 : Sum  OutDataType=sfix(16)  OutScaling=2^0  SaturateOnIntegerOverflow=on  InputSameDT=on  OutDataTypeStr=Inherit: Same as first input
  "c_alphaF " : Constant  Value=50000  OutDataType=sfix(16)  OutScaling=2^0
  n_F : Constant  Value=0.06  OutDataType=sfix(16)  OutScaling=2^0
  c_alphaF : Outport  OutDataType=sfix(16)  OutScaling=2^0
  delta_F : Outport  Port=2  OutDataType=sfix(16)  OutScaling=2^0
  wires:
  "      "/1 -> delta_F/1
  "c_alphaF "/1 -> "       "/1, c_alphaF/1
  n_F/1 -> "       "/3
  C_S/1 -> "       "/2
  Sum2/1 -> "      "/1
  Sum3/1 -> "      "/2
  "     "/1 -> Sum3/1
  1/ i_S/1 -> Sum2/1
  "   "/1 -> Sum2/2
  StWhlAngle/1 -> 1/ i_S/1
  "       "/1 -> "   "/1, Sum3/2
  beta + l_F * vYaw / v/1 -> "   "/2

== system SingleTrack_RTW/SingleTrack/single-track mass point model/yaw/sideslip angle/Subsystem ==
  vYaw : Inport
  v : Inport  Port=2
  In3 : Inport  Port=3
  If : If  IfExpression=u1 > 0.1 | u1 < -0.1
  If Action Subsystem : Subsystem  TreatAsAtomicUnit=on
  If Action Subsystem1 : Subsystem  TreatAsAtomicUnit=on
  Merge : Merge
  Sum1 : Sum  Inputs=-+  OutDataType=sfix(16)  OutScaling=2^0  SaturateOnIntegerOverflow=on  InputSameDT=on  OutDataTypeStr=Inherit: Same as first input
  Out1 : Outport
  wires:
  vYaw/1 -> Sum1/1
  v/1 -> If Action Subsystem/1(v), If/1
  Sum1/1 -> Out1/1
  If Action Subsystem/1(Out1) -> Merge/1
  If Action Subsystem1/1(Out1) -> Merge/2
  Merge/1 -> Sum1/2
  If/2 -> If Action Subsystem1/Action
  In3/1 -> If Action Subsystem/2(In3)
  If/1 -> If Action Subsystem/Action

== system SingleTrack_RTW/SingleTrack/single-track mass point model/yaw/side forces/Subsystem/If Action Subsystem ==
  v : Inport
  vYaw : Inport  Port=2
  Action Port : ActionPort  ActionType=then
  vYaw / v : Product  Inputs=/*  OutDataType=sfix(16)  OutScaling=2^0  SaturateOnIntegerOverflow=on  InputSameDT=on  OutDataTypeStr=Inherit: Same as first input
  Out1 : Outport  OutDataType=sfix(16)  OutScaling=2^0  InitialOutput=0
  wires:
  v/1 -> vYaw / v/1
  vYaw/1 -> vYaw / v/2
  vYaw / v/1 -> Out1/1

== system SingleTrack_RTW/SingleTrack/single-track mass point model/yaw/side forces/Subsystem/If Action Subsystem1 ==
  Action Port : ActionPort  ActionType=else
  Constant : Constant  Value=0  OutDataType=sfix(16)  OutScaling=2^0
  Out1 : Outport  OutDataType=sfix(16)  OutScaling=2^0  InitialOutput=0
  wires:
  Constant/1 -> Out1/1

== system SingleTrack_RTW/SingleTrack/single-track mass point model/yaw/sideslip angle/Subsystem/If Action Subsystem ==
  v : Inport
  In3 : Inport  Port=2
  Action Port : ActionPort  ActionType=then
  "    " : Product  Inputs=/*  OutDataType=sfix(16)  OutScaling=2^0  SaturateOnIntegerOverflow=on  InputSameDT=on  OutDataTypeStr=Inherit: Same as first input
  Out1 : Outport  OutDataType=sfix(16)  OutScaling=2^0  InitialOutput=0
  wires:
  v/1 -> "    "/1
  In3/1 -> "    "/2
  "    "/1 -> Out1/1

== system SingleTrack_RTW/SingleTrack/single-track mass point model/yaw/sideslip angle/Subsystem/If Action Subsystem1 ==
  Action Port : ActionPort  ActionType=else
  Constant : Constant  Value=0  OutDataType=sfix(16)  OutScaling=2^0
  Out1 : Outport  OutDataType=sfix(16)  OutScaling=2^0  InitialOutput=0
  wires:
  Constant/1 -> Out1/1
